simulink model "Closed_loop"  (R2024b)
settings: Solver=VariableStepAuto  StartTime=0.0  StopTime=10.0  RelTol=1e-3
values from neighbouring files (symbols this model uses):
  A = 3    [closed_loop_code.m]
  F = 1    [PID_Controlled_SPD_run.m]    (also in closed_loop_code.m = 2; run_SMD_Laplace.m; run_Spring_mass_Damper.m = 10)
  Ti = 0.5    [closed_loop_code.m]
settings Model: Creator=sajim  LastModifiedBy=sajim

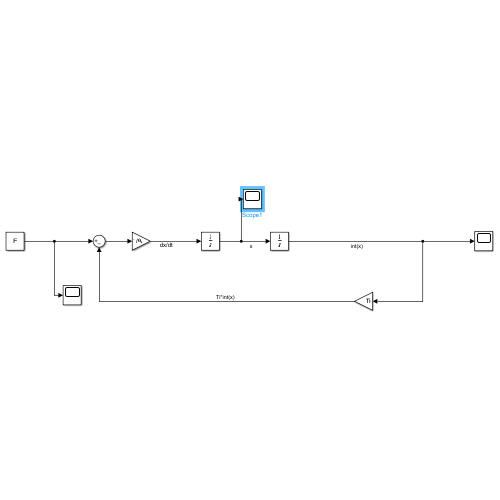
[thumbnail: Simulink's stored preview of the top-level diagram]
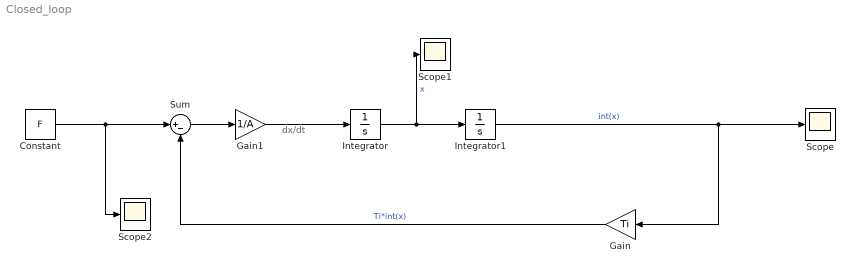
== system Closed_loop ==
  note: dx/dt
  Constant : Constant  Value=F
  Gain : Gain  Gain=Ti
  Gain1 : Gain  Gain=1/A
  Integrator : Integrator
  Integrator1 : Integrator
  Scope : Scope
  Scope1 : Scope
  Scope2 : Scope
  Sum : Sum  Inputs=|+-
  wires:
  Integrator/1 -> Scope1/1, Integrator1/1  "x"
  Integrator1/1 -> Scope/1, Gain/1  "int(x)"
  Gain/1 -> Sum/2  "Ti*int(x)"
  Constant/1 -> Scope2/1, Sum/1
  Sum/1 -> Gain1/1
  Gain1/1 -> Integrator/1
